simulink model "Local_linearization"  (R2016b)
settings: Solver=VariableStepAuto  StartTime=0.0  StopTime=10.0  RelTol=1e-3
settings Model: Creator=liana  LastModifiedBy=liana

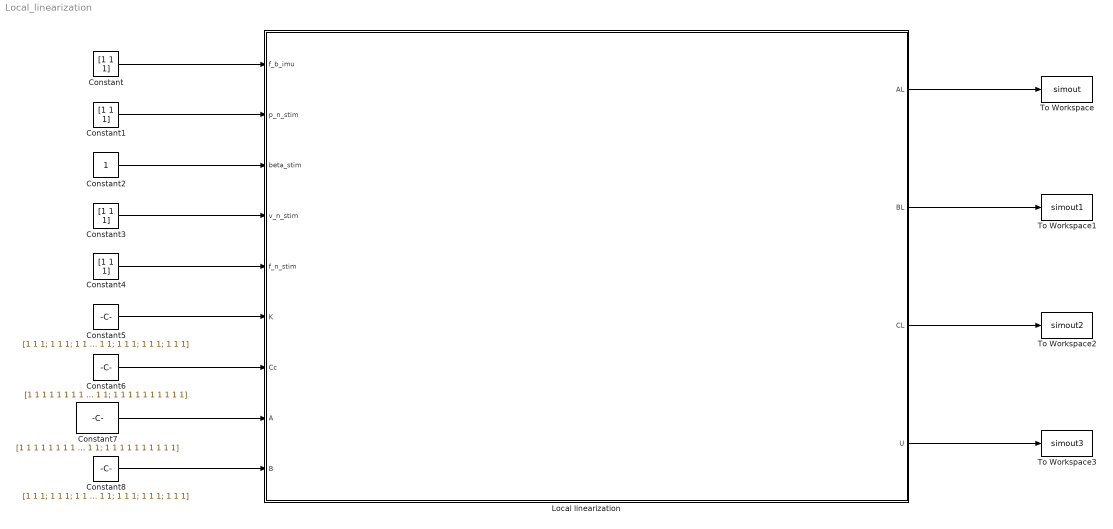
== system Local_linearization ==
  Constant{,1,3..4} (4 alike) : Constant  Value=[1 1 1]
  Constant2 : Constant
  Constant5 : Constant  Value=[1 1 1; 1 1 1; 1 1 1; 1 1 1; 1 1 1; 1 1 1; 1 1 1; 1 1 1; 1 1 1; 1 1 1]
  Constant6 : Constant  Value=[1 1 1 1 1 1 1 1 1 1; 1 1 1 1 1 1 1 1 1 1; 1 1 1 1 1 1 1 1 1 1]
  Constant7 : Constant  Value=[1 1 1 1 1 1 1 1 1 1; 1 1 1 1 1 1 1 1 1 1; 1 1 1 1 1 1 1 1 1 1; 1 1 1 1 1 1 1 1 1 1; 1 1 1 1 1 1 1 1 1 1; 1 1 1 1 1 1 1 1 1 1; 1 1 1 1 1 1 1 1 1 1; 1 1 1 1 1 1 1 1 1 1; 1 1 1 1 1 1 1 1 1 1; 1 1 1 1 1 1 1 1 1 1]
  Constant8 : Constant  Value=[1 1 1; 1 1 1; 1 1 1; 1 1 1; 1 1 1; 1 1 1; 1 1 1; 1 1 1; 1 1 1; 1 1 1]
  Local linearization : Subsystem
  To Workspace : ToWorkspace  VariableName=simout  SampleTime=-1
  To Workspace1 : ToWorkspace  VariableName=simout1  SampleTime=-1
  To Workspace2 : ToWorkspace  VariableName=simout2  SampleTime=-1
  To Workspace3 : ToWorkspace  VariableName=simout3  SampleTime=-1
  wires:
  Constant/1 -> Local linearization/1(f_b_imu)
  Constant1/1 -> Local linearization/2(p_n_stim)
  Constant2/1 -> Local linearization/3(beta_stim)
  Constant4/1 -> Local linearization/5(f_n_stim)
  Constant3/1 -> Local linearization/4(v_n_stim)
  Constant5/1 -> Local linearization/6(K)
  Constant6/1 -> Local linearization/7(Cc)
  Constant7/1 -> Local linearization/8(A)
  Constant8/1 -> Local linearization/9(B)
  Local linearization/1(AL) -> To Workspace/1
  Local linearization/2(BL) -> To Workspace1/1
  Local linearization/3(CL) -> To Workspace2/1
  Local linearization/4(U) -> To Workspace3/1

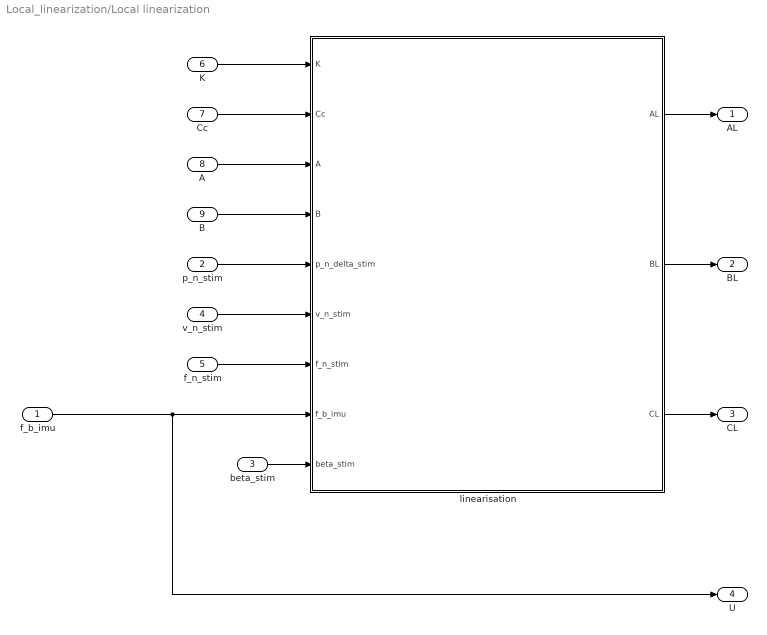
== system Local_linearization/Local linearization ==
  f_b_imu : Inport
  p_n_stim : Inport  Port=2
  beta_stim : Inport  Port=3
  v_n_stim : Inport  Port=4
  f_n_stim : Inport  Port=5
  K : Inport  Port=6
  Cc : Inport  Port=7
  A : Inport  Port=8
  B : Inport  Port=9
  linearisation : MATLAB Function  TreatAsAtomicUnit=on
  AL : Outport
  BL : Outport  Port=2
  CL : Outport  Port=3
  U : Outport  Port=4
  wires:
  linearisation/1(AL) -> AL/1
  linearisation/2(BL) -> BL/1
  linearisation/3(CL) -> CL/1
  K/1 -> linearisation/1(K)
  Cc/1 -> linearisation/2(Cc)
  A/1 -> linearisation/3(A)
  B/1 -> linearisation/4(B)
  p_n_stim/1 -> linearisation/5(p_n_delta_stim)
  beta_stim/1 -> linearisation/9(beta_stim)
  f_n_stim/1 -> linearisation/7(f_n_stim)
  v_n_stim/1 -> linearisation/6(v_n_stim)
  f_b_imu/1 -> U/1, linearisation/8(f_b_imu)

== matlab function Local_linearization/Local linearization/linearisation ==
  data: K input size=[10,3]; AL output size=[10,10]; BL output size=[10,3]; CL output size=[3,10]; Cc input size=[3,10]; A input size=[10,10]; B input size=[10,3]; p_n_delta_stim input size=[1,3]; v_n_stim input size=[1,3]; f_n_stim input size=[1,3]; f_b_imu input size=[1,3]; beta_stim input size=1
function [AL, BL, CL] = linearisation(K,Cc,A,B, p_n_delta_stim, v_n_stim, f_n_stim, f_b_imu, beta_stim)

 % building state vector
 % xsi = [p_n_stim ; beta_stim; v_n_stim; f_n_tim];
%   xsi = zeros(10,1);
%   xsi(1:3,1) = p_n_delta_stim;
%   xsi(4,1) = beta_stim;
%   xsi(5:7,1) = v_n_stim;
%   xsi(8:10,1) = f_n_stim;
 % coder.extrinsic('ss');
 % sys = ss(A-K*C,B,C,0);
% % getting work point
%coder.extrinsic('trim');
%[X,U,Y,DX] = trim('sys', xsi);

% computing linearisation model
%coder.extrinsic('linmod');
%[AL, BL, CL, DL] = linmod('sys',X,U);

  
AL = zeros(10,10);
BL = zeros(10,3);
CL = zeros(3, 10);


coder.extrinsic('LinearizationFun');

[Al,Bl,Cl] = LinearizationFun(K,Cc,A,B);

p_n0 = p_n_delta_stim(1, 1);
p_n1 = p_n_delta_stim (1,2);
p_n2 = p_n_delta_stim(1,3);

v_n0 = v_n_stim(1, 1);
v_n1 = v_n_stim(1,2);
v_n2 = v_n_stim(1,3);

f_n0 = f_n_stim(1,1);
f_n1 = f_n_stim(1,2);
f_n2 = f_n_stim(1,3);

f_b0 = f_b_imu(1,1);
f_b1 = f_b_imu(1,2);
f_b2 = f_b_imu(1,3);


coder.extrinsic('eval');

AL_ = eval(Al);
BL_ = eval(Bl);
CL_ = eval(Cl);

% AL_ = feval('Al', p_n0, p_n1, p_n2,v_n0, v_n1, v_n2, f_n0, f_n1, f_n2, beta_stim);
% BL_ = feval('Bl', f_b0, f_b1, f_b2);
% CL_ = feval('Cl', p_n0, p_n1, p_n2,v_n0, v_n1, v_n2, f_n0, f_n1, f_n2, beta_stim);
% 

AL = AL_;
BL = BL_;
CL = CL_;


end
